simulink model "PROBA2mdl_Chapter3"  (R2022b)
settings: Solver=ode45  StartTime=0.0  StopTime=T  MaxStep=0.1  RelTol=1e-6  EnableMultiTasking=on
undefined symbols (not defined in the file): J_2, mu, r_I_ini, rE, v_I_ini
settings Model: Creator=Steve  LastModifiedBy=boaza
settings SolverCC: AlgebraicLoopSolver=TrustRegion
settings DataIOCC: LimitDataPoints=on  SaveFormat=Array  ReturnWorkspaceOutputs=off
settings OptimizationCC: ExpressionDepthLimit=2147483647  LifeSpan=inf
settings DebuggingCC: UnderspecifiedInitializationDetection=Classic  MergeDetectMultiDrivingBlocksExec=none  SolverPrmCheckMsg=warning  UnconnectedInputMsg=warning  UnconnectedOutputMsg=warning  UnconnectedLineMsg=warning  AllowSymbolicDim=off  StateNameClashWarn=warning  SFUnexpectedBacktrackingDiag=warning  SFNoUnconditionalDefaultTransitionDiag=warning  SFMachineParentedDataDiag=warning  ArithmeticOperatorsInVariantConditions=warning
settings HardwareCC: ProdBitPerPointer=32  ProdBitPerSizeT=32  ProdBitPerPtrDiffT=32  ProdLargestAtomicFloat=None  ProdIntDivRoundTo=Undefined  ProdEndianess=Unspecified  ProdWordSize=32  ProdHWDeviceType=32-bit Generic
settings ModelReferenceCC: EnableRefExpFcnMdlSchedulingChecks=on  PropagateSignalLabelsOutOfModel=off
settings SFSimCC: SimUseLocalCustomCode=off  CustomCodeUndefinedFunction=UseInterfaceOnly
settings RTWCC: RTWUseLocalCustomCode=off  DLArmComputeVersion=19.05
settings CodeAppCC: StateflowObjectComments=on
settings GRTTargetCC: TargetLangStandard=C89/C90 (ANSI)
settings ConfigComp: CovMetricSettings=dw  CovSaveCumulativeToWorkspaceVar=on  CovSaveSingleToWorkspaceVar=on  CovExternalEMLEnable=off  CovSFcnEnable=off

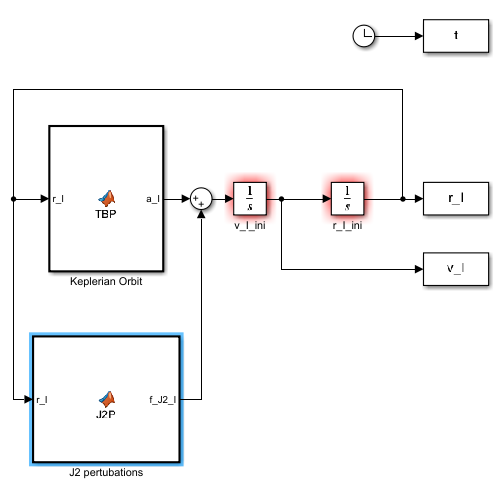
[thumbnail: Simulink's stored preview of the top-level diagram]
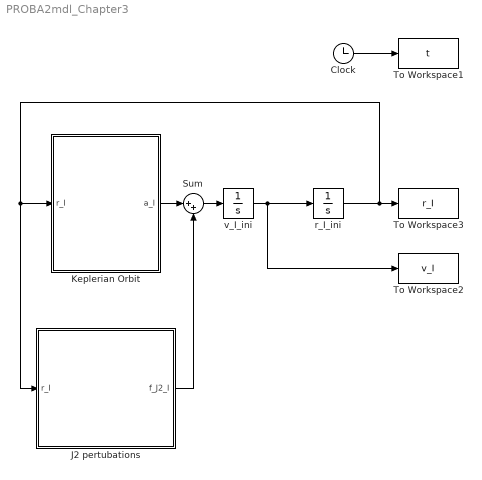
== system PROBA2mdl_Chapter3 ==
  Clock : Clock
  J2 pertubations : MATLAB Function  TreatAsAtomicUnit=on
  Keplerian Orbit : MATLAB Function  TreatAsAtomicUnit=on
  Sum : Sum  Inputs=|++
  To Workspace1 : ToWorkspace  VariableName=t  SampleTime=-1
  To Workspace2 : ToWorkspace  VariableName=v_I  SampleTime=-1
      settings: Save2DSignal=2-D array (concatenate along first dimension)
  To Workspace3 : ToWorkspace  VariableName=r_I  SampleTime=-1
      settings: Save2DSignal=2-D array (concatenate along first dimension)
  r_I_ini : Integrator  InitialCondition=r_I_ini
  v_I_ini : Integrator  InitialCondition=v_I_ini
  wires:
  r_I_ini/1 -> To Workspace3/1, J2 pertubations/1(r_I), Keplerian Orbit/1(r_I)
  v_I_ini/1 -> To Workspace2/1, r_I_ini/1
  Clock/1 -> To Workspace1/1
  J2 pertubations/1(f_J2_I) -> Sum/2
  Keplerian Orbit/1(a_I) -> Sum/1
  Sum/1 -> v_I_ini/1

== matlab function PROBA2mdl_Chapter3/J2 pertubations ==
  data: f_J2_I output; rE parameter; J_2 parameter; mu parameter; r_I input
function f_J2_I =  J2P(rE, J_2, mu, r_I)

f_J2_I = 3*mu*J_2*rE^2/(2*(norm(r_I)^5))...
    *(...
    (5*(r_I(3)^2)/(norm(r_I)^2)-1)*r_I - 2*[0; 0; r_I(3)]...
    );

end

== matlab function PROBA2mdl_Chapter3/Keplerian Orbit ==
  data: r_I input; mu parameter; a_I output
function  a_I =  TBP(r_I, mu)

% ---------------------------------------------------------------
% TBP
% ---------------------------------------------------------------
% Description:
% Compute the spacecraft acceleration in ECI, using the two-body
% equation of motion.
% ---------------------------------------------------------------
% Inputs:
% r_I => components of r in ECI (3 x 1 matrix)
% ---------------------------------------------------------------
% Outputs:
% a_I => components of the acceleration in ECI (3 x 1 matrix)
% ---------------------------------------------------------------
% Parameters:
% mu => gravitational constant of the Earth
% ---------------------------------------------------------------
% Copyright:
% Steve Ulrich, 2014 
% ---------------------------------------------------------------

% Compute orbital radius
rmod = sqrt( r_I(1)*r_I(1) + r_I(2)*r_I(2) + r_I(3)*r_I(3) );

% Spacecraft acceleration
a_I = -mu/rmod^3*r_I;
end
